simulink model "model25r"  (R2020b)
settings: Solver=VariableStepAuto  StartTime=0.0  StopTime=120  RelTol=1e-3
libraries: fuzblock x1
settings Model: Creator=chico  LastModifiedBy=chico

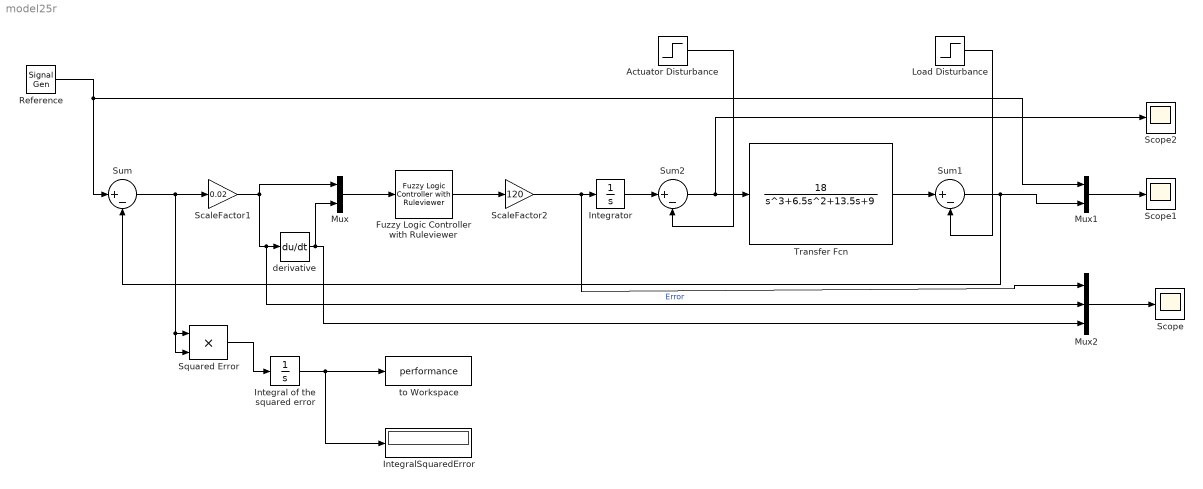
== system model25r ==
  Actuator Disturbance : Step  Time=40  After=0  SampleTime=0
  Fuzzy Logic Controller with Ruleviewer : fuzblock/Fuzzy Logic  Controller  with Ruleviewer  fismatrix=fis  Ts=2
  Integral of the squared error : Integrator
  IntegralSquaredError : Display
  Integrator : Integrator
  Load Disturbance : Step  Time=80  After=0  SampleTime=0
  Mux : Mux  Inputs=2
  Mux1 : Mux  Inputs=2
  Mux2 : Mux  Inputs=3
  Reference : SignalGenerator  Frequency=0.5  Units=rad/sec
  ScaleFactor1 : Gain  Gain=0.02
  ScaleFactor2 : Gain  Gain=120
  Scope : Scope
  Scope1 : Scope
  Scope2 : Scope
  Squared Error : Product
  Sum : Sum  Inputs=|+-
  Sum1 : Sum  Inputs=|+-
  Sum2 : Sum  Inputs=|+-
  Transfer Fcn : TransferFcn  Numerator=[18]  Denominator=[1 6.5 13.5 9]
  derivative : Derivative
  to Workspace : ToWorkspace  VariableName=performance  SaveFormat=Timeseries  SampleTime=-1
  wires:
  Sum/1 -> Squared Error/2, Squared Error/1, ScaleFactor1/1
  Reference/1 -> Sum/1, Mux1/1
  ScaleFactor1/1 -> Mux/1, Mux2/2, derivative/1  "Error"
  derivative/1 -> Mux/2, Mux2/3
  Fuzzy Logic Controller with Ruleviewer/1 -> ScaleFactor2/1
  ScaleFactor2/1 -> Mux2/1, Integrator/1
  Integrator/1 -> Sum2/1
  Sum2/1 -> Scope2/1, Transfer Fcn/1
  Actuator Disturbance/1 -> Sum2/2
  Load Disturbance/1 -> Sum1/2
  Mux1/1 -> Scope1/1
  Sum1/1 -> Mux1/2, Sum/2
  Mux2/1 -> Scope/1
  Squared Error/1 -> Integral of the squared error/1
  Integral of the squared error/1 -> IntegralSquaredError/1, to Workspace/1
  Mux/1 -> Fuzzy Logic Controller with Ruleviewer/1
  Transfer Fcn/1 -> Sum1/1
